simulink model "Task_M_mod"  (R2018a)
settings: Solver=ode4  StartTime=0.0  StopTime=10.0  FixedStep=0.01  RelTol=1e-3  EnableMultiTasking=on
values from neighbouring files (symbols this model uses):
  a0 = 1    [task_B_scr.m]    (also in task_E_scr.m = 0.5; task_H_real_scr.m = 0.5; task_H_scr.m = 0.5; task_J_scr.m = 0.5)
  a1 = 0.5    [task_D_scr.m]    (also in task_M_scr.m; task_N_scr.m = 1)
  b0 = 2    [task_B_scr.m]    (also in task_C_scr.m; task_D_scr.m; task_E_scr.m = 1; task_G_scr.m)
  wr = 0.025; sim('Task_J_mod',tfin)    [task_J_scr.m]    (also in task_L_scr.m = 0.01; sim('Task_L_mod',tfin); task_M_scr.m = 0.005; sim('Task_M_mod',tfin))
libraries: simulink x2
settings Model: Creator=Yurii  LastModifiedBy=Master
settings DataIOCC: LimitDataPoints=on  SaveFormat=Array
settings OptimizationCC: LifeSpan=inf
settings DebuggingCC: UnderspecifiedInitializationDetection=Classic  MergeDetectMultiDrivingBlocksExec=none  SolverPrmCheckMsg=warning  SFUnexpectedBacktrackingDiag=warning  SFNoUnconditionalDefaultTransitionDiag=warning  SFExecutionAtInitializationDiag=none
settings HardwareCC: ProdBitPerPointer=32  ProdBitPerSizeT=32  ProdBitPerPtrDiffT=32  ProdLargestAtomicFloat=None  ProdIntDivRoundTo=Undefined  ProdEndianess=Unspecified  ProdWordSize=32  ProdHWDeviceType=32-bit Generic
settings ModelReferenceCC: PropagateSignalLabelsOutOfModel=off
settings CodeAppCC: StateflowObjectComments=on
settings GRTTargetCC: TargetLangStandard=C89/C90 (ANSI)  GeneratePreprocessorConditionals=Disable all
settings ConfigComp: CovMetricSettings=dw  CovHtmlReporting=on  CovSaveCumulativeToWorkspaceVar=on  CovSaveSingleToWorkspaceVar=on  CovExternalEMLEnable=off

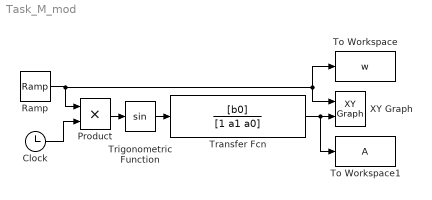
== system Task_M_mod ==
  Clock : Clock
  Product : Product
  Ramp : simulink/Sources/Ramp  slope=wr  start=0  InitialOutput=0
  To Workspace : ToWorkspace  VariableName=w  SaveFormat=Timeseries  SampleTime=-1
  To Workspace1 : ToWorkspace  VariableName=A  SaveFormat=Timeseries  SampleTime=-1
  Transfer Fcn : TransferFcn  Numerator=[b0]  Denominator=[1 a1 a0]
  Trigonometric Function : Trigonometry
  XY Graph : simulink/Sinks/XY Graph  xmin=0  xmax=3  ymin=-2  ymax=2  st=0
  wires:
  Product/1 -> Trigonometric Function/1
  Transfer Fcn/1 -> XY Graph/2, To Workspace1/1
  Clock/1 -> Product/2
  Ramp/1 -> XY Graph/1, To Workspace/1, Product/1
  Trigonometric Function/1 -> Transfer Fcn/1
